simulink model "project"  (R2020b)
settings: Solver=VariableStepAuto  StartTime=0.0  StopTime=inf  RelTol=1e-3
libraries: simulink x1
settings Model: Creator=99003727  LastModifiedBy=99003727

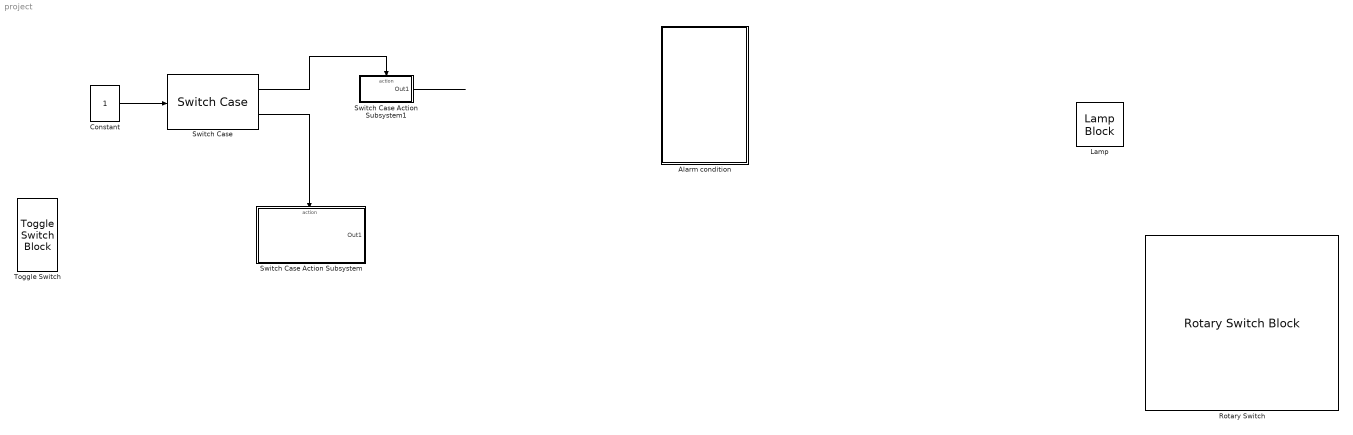
== system project ==
  Alarm condition : Subsystem
  Constant : Constant
  Lamp : LampBlock
  Rotary Switch : RotarySwitchBlock
      settings: Values={{'SlowFlash', 'nope', 'Fastflash', 'Solid'}, [0 1 2 3]}
  Switch Case : SwitchCase  CaseConditions={0,1}  ShowDefaultCase=off
  Switch Case Action Subsystem : Subsystem  TreatAsAtomicUnit=on
  Switch Case Action Subsystem1 : Subsystem  TreatAsAtomicUnit=on
  Toggle Switch : ToggleSwitchBlock
      settings: Values={{'Off', 'On'}, [0 1]}
  wires:
  Constant/1 -> Switch Case/1
  Switch Case/2 -> Switch Case Action Subsystem/Action
  Switch Case/1 -> Switch Case Action Subsystem1/Action
  Switch Case Action Subsystem1/1(Out1) -> ?

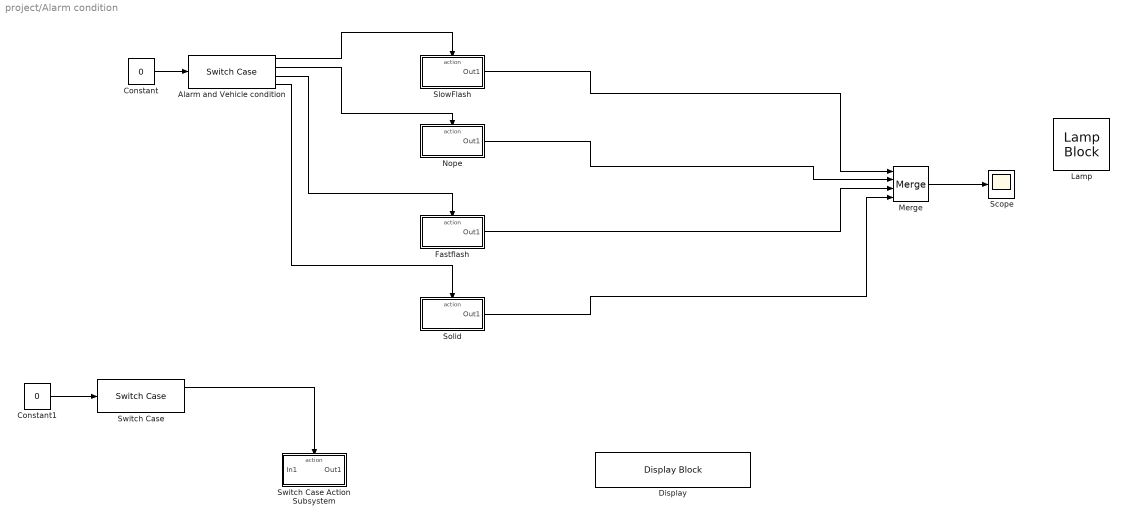
== system project/Alarm condition ==
  Alarm and Vehicle condition : SwitchCase  CaseConditions={0,1,2,3}  ShowDefaultCase=off
  Constant : Constant  Value=0
  Constant1 : Constant  Value=0
  Display : DisplayBlock  LabelPosition=Hide  Format=short  Transparency=1
  Fastflash : Subsystem  TreatAsAtomicUnit=on
  Lamp : LampBlock
  Merge : Merge  Inputs=4
  Nope : Subsystem  TreatAsAtomicUnit=on
  Scope : Scope
  SlowFlash : Subsystem  TreatAsAtomicUnit=on
  Solid : Subsystem  TreatAsAtomicUnit=on
  Switch Case : SwitchCase  CaseConditions={0,1}  ShowDefaultCase=off
  Switch Case Action Subsystem : Subsystem  TreatAsAtomicUnit=on
  wires:
  Nope/1(Out1) -> Merge/2
  SlowFlash/1(Out1) -> Merge/1
  Fastflash/1(Out1) -> Merge/3
  Solid/1(Out1) -> Merge/4
  Merge/1 -> Scope/1
  Alarm and Vehicle condition/1 -> SlowFlash/Action
  Alarm and Vehicle condition/2 -> Nope/Action
  Alarm and Vehicle condition/3 -> Fastflash/Action
  Alarm and Vehicle condition/4 -> Solid/Action
  Constant/1 -> Alarm and Vehicle condition/1
  Switch Case/1 -> Switch Case Action Subsystem/Action
  Constant1/1 -> Switch Case/1

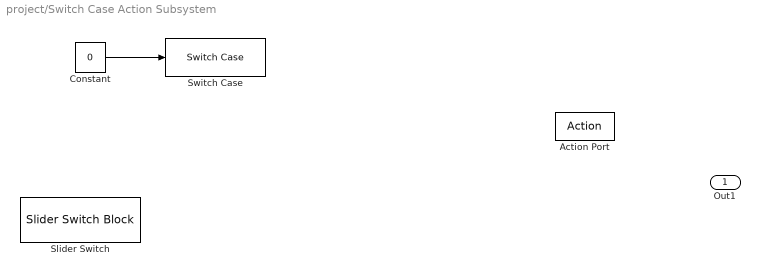
== system project/Switch Case Action Subsystem ==
  Action Port : ActionPort  ActionPortLabel=case [ 1 ]:
  Constant : Constant  Value=0
  Slider Switch : SliderSwitchBlock
      settings: Values={{'Off', 'On'}, [0 1]}
  Switch Case : SwitchCase  CaseConditions={1,2}  ShowDefaultCase=off
  Out1 : Outport
  wires:
  ? -> Out1/1
  Constant/1 -> Switch Case/1

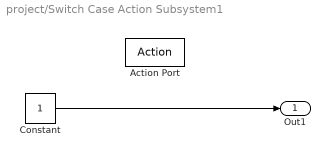
== system project/Switch Case Action Subsystem1 ==
  Action Port : ActionPort  ActionPortLabel=case [ 0 ]:
  Constant : Constant
  Out1 : Outport
  wires:
  Constant/1 -> Out1/1

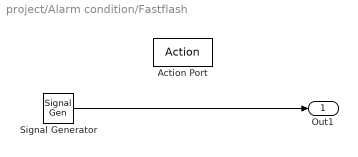
== system project/Alarm condition/Fastflash ==
  Action Port : ActionPort  ActionPortLabel=case [ 2 ]:
  Signal Generator : SignalGenerator  WaveForm=square  Frequency=20
  Out1 : Outport
  wires:
  Signal Generator/1 -> Out1/1

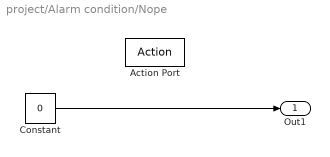
== system project/Alarm condition/Nope ==
  Action Port : ActionPort  ActionPortLabel=case [ 1 ]:
  Constant : Constant  Value=0
  Out1 : Outport
  wires:
  Constant/1 -> Out1/1

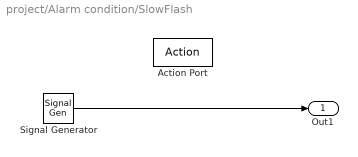
== system project/Alarm condition/SlowFlash ==
  Action Port : ActionPort  ActionPortLabel=case [ 0 ]:
  Signal Generator : SignalGenerator  WaveForm=square  Frequency=0.0005
  Out1 : Outport
  wires:
  Signal Generator/1 -> Out1/1

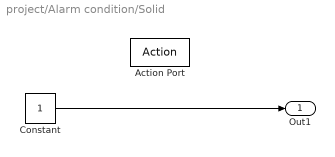
== system project/Alarm condition/Solid ==
  Action Port : ActionPort  ActionPortLabel=case [ 3 ]:
  Constant : Constant
  Out1 : Outport
  wires:
  Constant/1 -> Out1/1

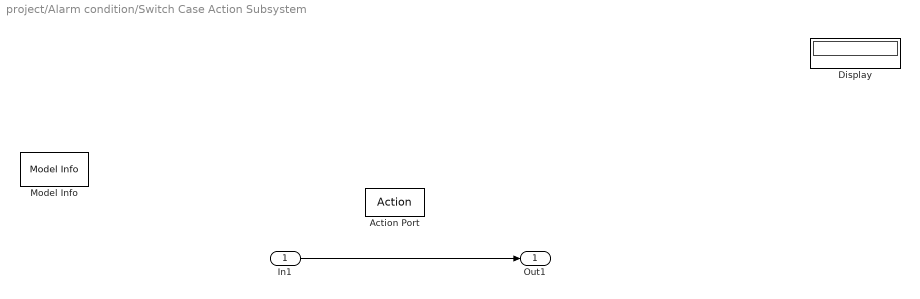
== system project/Alarm condition/Switch Case Action Subsystem ==
  In1 : Inport
  Action Port : ActionPort  ActionPortLabel=case [ 1 ]:
  Display : Display
  Model Info : simulink/Model-Wide Utilities/Model Info  Frame=on  DisplayStringWithTags=Engine is OFF  HorizontalTextAlignment=Center  LeftAlignmentValue=0.5
  Out1 : Outport
  wires:
  In1/1 -> Out1/1
